simulink subsystem "SMC_mathmatical"  (R2023a)
settings: Solver=VariableStepAuto  StartTime=0.0  StopTime=10.0  RelTol=1e-3
settings Model: Creator=hollis  LastModifiedBy=ethan

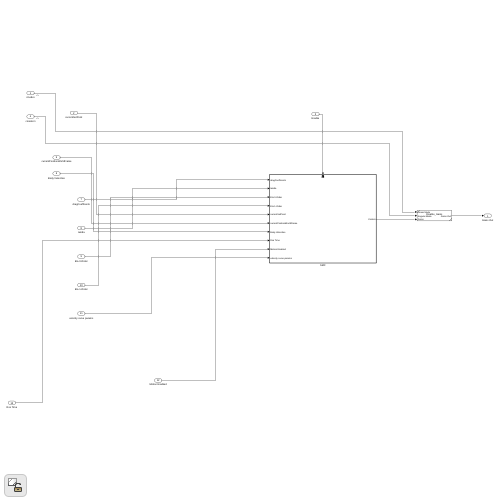
[thumbnail: Simulink's stored preview of the top-level diagram]
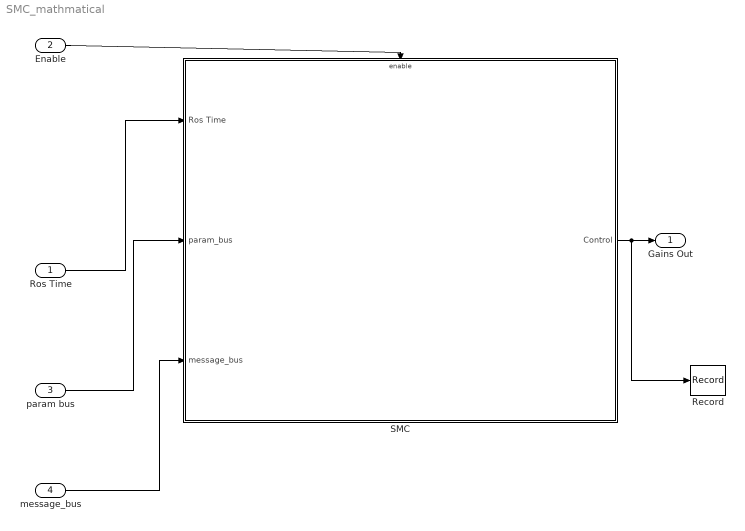
== system SMC_mathmatical ==
  Ros Time : Inport
  Enable : Inport  Port=2
  param bus : Inport  Port=3
  message_bus : Inport  Port=4
  Record : Record  FileSettingsInternal="{\"entries\":[{\"content\":{\"excelSettings\":{\"content\":{},\"type\":\"Streamout.ExcelSettings\"}},\"type\":\"Streamout.FileSettingStorage\",\"uuid\":\"\"}],\"packageUris\":[\"http:\\/\\/schema.mathworks.com\\/mf0\\/streamout_blocks\\/R2020a\"],\"version\":\"1.0\"}"  Layout=[1 1]  SignalsInternal="{\"entries\":[{\"content\":{\"signals\":[{\"content\":{\"blockPath\":[],\"dimensions\":[6],\"domain\":\"\",\"hasChildren\":true,\"lineColor\":\"#22b573\",\"port\":1,\"signalID\":34895,\"signalName\":\"SMC\"},\"type\":\"RecordBlkView.Signal\",\"uuid\":\"\"},{\"content\":{\"blockPath\":[],\"channel\":[1],\"dimensions\":[6],\"domain\":\"\",\"lineColor\":\"#0072bd\",\"parentID\":34895,\"plots\":[1],\"port\":1,\"signalID\":34896,\"signalName\":\"SMC\"},\"type\":\"RecordBlkView.Signal\",\"uuid\":\"\"},{\"content\":{\"blockPath\":[],\"channel\":[2],\"dimensions\":[6],\"domain\":\"\",\"lineColor\":\"#a2142f\",\"parentID\":34895,\"plots\":[1],\"port\":1,\"signalID\":34897,\"signalName\":\"SMC\"},\"type\":\"RecordBlkView.Signal\",\"uuid\":\"\"},{\"content\":{\"blockPath\":[],\"channel\":[3],\"dimensions\":[6],\"domain\":\"\",\"lineColor\":\"#139fff\",\"parentID\":34895,\"plots\":[1],\"port\":1,\"signalID\":34898,\"signalName\":\"SMC\"},\"type\":\"RecordBlkView.Signal\",\"uuid\":\"\"},{\"content\":{\"blockPath\":[],\"channel\":[4],\"dimensions\":[6],\"domain\":\"\",\"lineColor\":\"#ff6929\",\"parentID\":34895,\"plots\":[1],\"port\":1,\"signalID\":34899,\"signalName\":\"SMC\"},\"type\":\"RecordBlkView.Signal\",\"uuid\":\"\"},{\"content\":{\"blockPath\":[],\"channel\":[5],\"dimensions\":[6],\"domain\":\"\",\"lineColor\":\"#b746ff\",\"parentID\":34895,\"plots\":[1],\"port\":1,\"signalID\":34900,\"signalName\":\"SMC\"},\"type\":\"RecordBlkView.Signal\",\"uuid\":\"\"},{\"content\":{\"blockPath\":[],\"channel\":[6],\"dimensions\":[6],\"domain\":\"\",\"lineColor\":\"#64d413\",\"parentID\":34895,\"plots\":[1],\"port\":1,\"signalID\":34901,\"signalName\":\"SMC\"},\"type\":\"RecordBlkView.Signal\",\"uuid\":\"\"}]},\"type\":\"RecordBlkView.InputSignals\",\"uuid\":\"\"}],\"packageUris\":[\"http:\\/\\/schema.mathworks.com\\/mf0\\/streamout_blocks\\/R2020a\"],\"version\":\"1.0\"}"  VisualizationBindings="{\"sparklinesplugin\":{\"info\":[{\"bindingParametersList\":[],\"subplotID\":1}]}}"
  SMC : Subsystem
  Gains Out : Outport
  wires:
  SMC/1(Control) -> Gains Out/1, Record/1
  param bus/1 -> SMC/2(param_bus)
  Ros Time/1 -> SMC/1(Ros Time)
  Enable/1 -> SMC/Enable
  message_bus/1 -> SMC/3(message_bus)

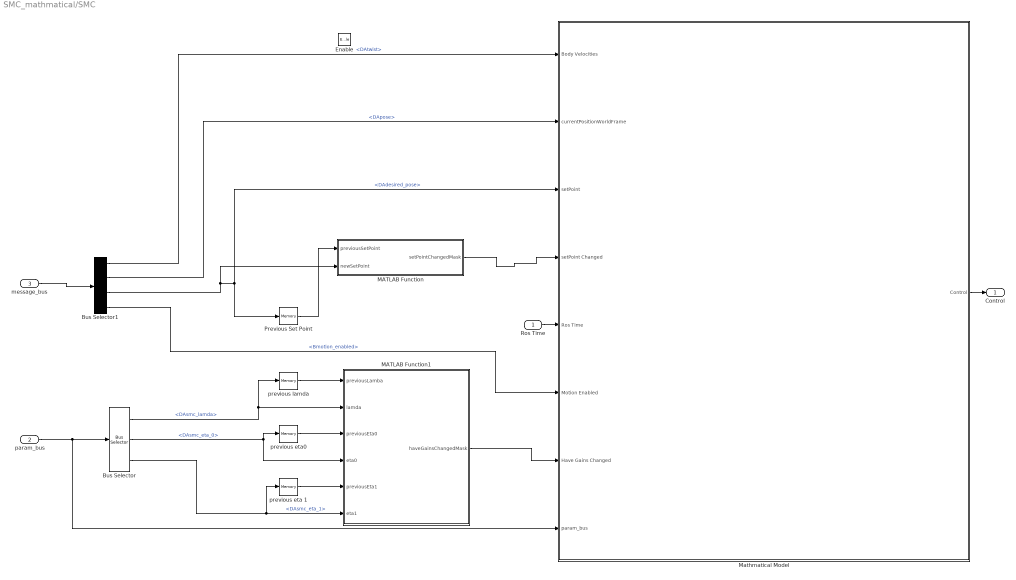
== system SMC_mathmatical/SMC ==
  Ros Time : Inport
  param_bus : Inport  Port=2
  message_bus : Inport  Port=3
  Enable : EnablePort
  Bus Selector : BusSelector  OutputSignals=DAsmc_lamda,DAsmc_eta_0,DAsmc_eta_1
  Bus Selector1 : BusSelector  OutputSignals=current_state.DAtwist,current_state.DApose,desired_pose.DAdesired_pose,Bmotion_enabled
  MATLAB Function : MATLAB Function  TreatAsAtomicUnit=on
  MATLAB Function1 : MATLAB Function  TreatAsAtomicUnit=on
  Mathmatical Model : Subsystem
  Previous Set Point : Memory  InitialCondition=[0,0,0,0,0,0,0]  InheritSampleTime=on
  previous eta 1 : Memory  InheritSampleTime=on
  previous eta0 : Memory  InheritSampleTime=on
  previous lamda : Memory  InheritSampleTime=on
  Control : Outport
  wires:
  Bus Selector1/1 -> Mathmatical Model/1(Body Velocities)  "<DAtwist>"
  Bus Selector1/2 -> Mathmatical Model/2(currentPositionWorldFrame)  "<DApose>"
  message_bus/1 -> Bus Selector1/1
  Bus Selector/3 -> MATLAB Function1/6(eta1), previous eta 1/1  "<DAsmc_eta_1>"
  Bus Selector/2 -> MATLAB Function1/4(eta0), previous eta0/1  "<DAsmc_eta_0>"
  Bus Selector/1 -> MATLAB Function1/2(lamda), previous lamda/1  "<DAsmc_lamda>"
  param_bus/1 -> Mathmatical Model/8(param_bus), Bus Selector/1
  MATLAB Function1/1(haveGainsChangedMask) -> Mathmatical Model/7(Have Gains Changed)
  previous eta 1/1 -> MATLAB Function1/5(previousEta1)
  previous eta0/1 -> MATLAB Function1/3(previousEta0)
  previous lamda/1 -> MATLAB Function1/1(previousLamba)
  Bus Selector1/4 -> Mathmatical Model/6(Motion Enabled)  "<Bmotion_enabled>"
  Ros Time/1 -> Mathmatical Model/5(Ros Time)
  Previous Set Point/1 -> MATLAB Function/1(previousSetPoint)
  MATLAB Function/1(setPointChangedMask) -> Mathmatical Model/4(setPoint Changed)
  Bus Selector1/3 -> Mathmatical Model/3(setPoint), Previous Set Point/1, MATLAB Function/2(newSetPoint)  "<DAdesired_pose>"
  Mathmatical Model/1(Control) -> Control/1

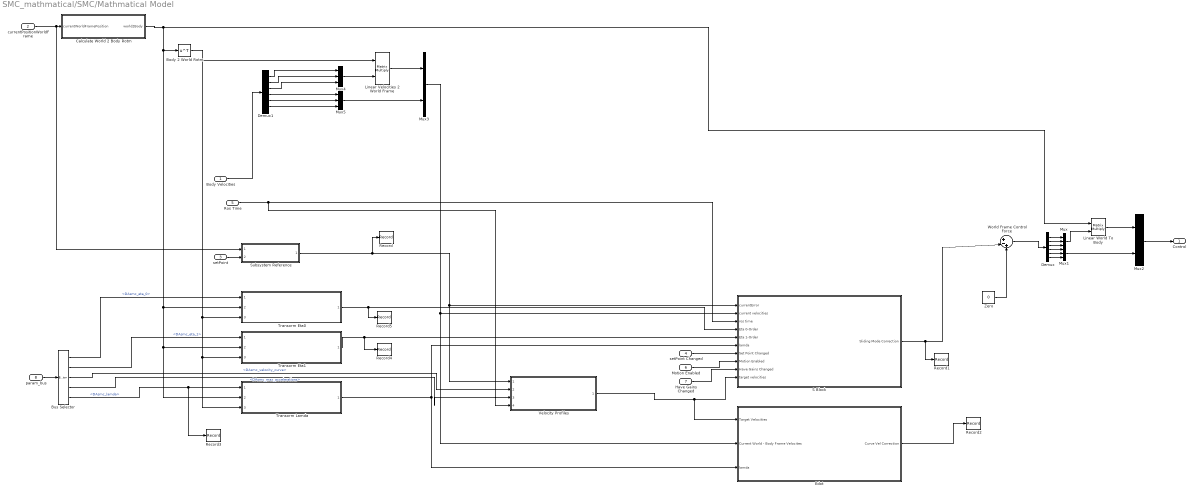
== system SMC_mathmatical/SMC/Mathmatical Model ==
  Body Velocities : Inport
  currentPositionWorldFrame : Inport  Port=2
  setPoint : Inport  Port=3
  setPoint Changed : Inport  Port=4
  Ros Time : Inport  Port=5
  Motion Enabled : Inport  Port=6
  Have Gains Changed : Inport  Port=7
  param_bus : Inport  Port=8
  Body 2 World Rotm : Math  Operator=transpose
  Bus Selector : BusSelector  OutputSignals=DAsmc_eta_0,DAsmc_eta_1,DAsmc_velocity_curve,DAsmc_max_accelerations,DAsmc_lamda
  Calculate World 2 Body Rotm : MATLAB Function  TreatAsAtomicUnit=on
  Demux : Demux  Outputs=6
  Demux1 : Demux  Outputs=6
  Edot : Subsystem
  Linear Velocities 2 World Frame : Product  Multiplication=Matrix(*)
  Linear World To Body : Product  Multiplication=Matrix(*)
  Mux{,1,4..5} (4 alike) : Mux  Inputs=3
  Mux2 : Mux  Inputs=2
  Mux3 : Mux  Inputs=2
  Record : Record  FileSettingsInternal="{\"entries\":[{\"content\":{\"excelSettings\":{\"content\":{},\"type\":\"Streamout.ExcelSettings\"}},\"type\":\"Streamout.FileSettingStorage\",\"uuid\":\"\"}],\"packageUris\":[\"http:\\/\\/schema.mathworks.com\\/mf0\\/streamout_blocks\\/R2020a\"],\"version\":\"1.0\"}"  Layout=[1 1]  SignalsInternal="{\"entries\":[{\"content\":{\"signals\":[{\"content\":{\"blockPath\":[],\"dimensions\":[1,6],\"domain\":\"\",\"hasChildren\":true,\"lineColor\":\"#0072bd\",\"port\":1,\"signalID\":34980,\"signalName\":\"Subsystem Reference\"},\"type\":\"RecordBlkView.Signal\",\"uuid\":\"\"},{\"content\":{\"blockPath\":[],\"channel\":[1,1],\"dimensions\":[1,6],\"domain\":\"\",\"lineColor\":\"#d95319\",\"parentID\":34980,\"plots\":[1],\"port\":1,\"signalID\":34981,\"signalName\":\"Subsystem Reference\"},\"type\":\"RecordBlkView.Signal\",\"uuid\":\"\"},{\"content\":{\"blockPath\":[],\"channel\":[1,2],\"dimensions\":[1,6],\"domain\":\"\",\"lineColor\":\"#b746ff\",\"parentID\":34980,\"plots\":[1],\"port\":1,\"signalID\":34982,\"signalName\":\"Subsystem Reference\"},\"type\":\"RecordBlkView.Signal\",\"uuid\":\"\"},{\"content\":{\"blockPath\":[],\"channel\":[1,3],\"dimensions\":[1,6],\"domain\":\"\",\"lineColor\":\"#64d413\",\"parentID\":34980,\"plots\":[1],\"port\":1,\"signalID\":34983,\"signalName\":\"Subsystem Reference\"},\"type\":\"RecordBlkView.Signal\",\"uuid\":\"\"},{\"content\":{\"blockPath\":[],\"channel\":[1,4],\"dimensions\":[1,6],\"domain\":\"\",\"lineColor\":\"#ff13a6\",\"parentID\":34980,\"plots\":[1],\"port\":1,\"signalID\":34984,\"signalName\":\"Subsystem Reference\"},\"type\":\"RecordBlkView.Signal\",\"uuid\":\"\"},{\"content\":{\"blockPath\":[],\"channel\":[1,5],\"dimensions\":[1,6],\"domain\":\"\",\"lineColor\":\"#fe330a\",\"parentID\":34980,\"plots\":[1],\"port\":1,\"signalID\":34985,\"signalName\":\"Subsystem Reference\"},\"type\":\"RecordBlkView.Signal\",\"uuid\":\"\"},{\"content\":{\"blockPath\":[],\"channel\":[1,6],\"dimensions\":[1,6],\"domain\":\"\",\"lineColor\":\"#22b573\",\"parentID\":34980,\"plots\":[1],\"port\":1,\"signalID\":34986,\"signalName\":\"Subsystem Reference\"},\"type\":\"RecordBlkView.Signal\",\"uuid\":\"\"}]},\"type\":\"RecordBlkView.InputSignals\",\"uuid\":\"\"}],\"packageUris\":[\"http:\\/\\/schema.mathworks.com\\/mf0\\/streamout_blocks\\/R2020a\"],\"version\":\"1.0\"}"  VisualizationBindings="{\"sparklinesplugin\":{\"info\":[{\"bindingParametersList\":[],\"subplotID\":1}]}}"
  Record1 : Record  FileSettingsInternal="{\"entries\":[{\"content\":{\"excelSettings\":{\"content\":{},\"type\":\"Streamout.ExcelSettings\"}},\"type\":\"Streamout.FileSettingStorage\",\"uuid\":\"\"}],\"packageUris\":[\"http:\\/\\/schema.mathworks.com\\/mf0\\/streamout_blocks\\/R2020a\"],\"version\":\"1.0\"}"  Layout=[1 1]  SignalsInternal="{\"entries\":[{\"content\":{\"signals\":[{\"content\":{\"blockPath\":[],\"dimensions\":[6,1],\"domain\":\"\",\"hasChildren\":true,\"lineColor\":\"#22b573\",\"port\":1,\"signalID\":34997,\"signalName\":\"S Block\"},\"type\":\"RecordBlkView.Signal\",\"uuid\":\"\"},{\"content\":{\"blockPath\":[],\"channel\":[1,1],\"dimensions\":[6,1],\"domain\":\"\",\"lineColor\":\"#0072bd\",\"parentID\":34997,\"plots\":[1],\"port\":1,\"signalID\":34998,\"signalName\":\"S Block\"},\"type\":\"RecordBlkView.Signal\",\"uuid\":\"\"},{\"content\":{\"blockPath\":[],\"channel\":[2,1],\"dimensions\":[6,1],\"domain\":\"\",\"lineColor\":\"#4dbeee\",\"parentID\":34997,\"plots\":[1],\"port\":1,\"signalID\":34999,\"signalName\":\"S Block\"},\"type\":\"RecordBlkView.Signal\",\"uuid\":\"\"},{\"content\":{\"blockPath\":[],\"channel\":[3,1],\"dimensions\":[6,1],\"domain\":\"\",\"lineColor\":\"#a2142f\",\"parentID\":34997,\"plots\":[1],\"port\":1,\"signalID\":35000,\"signalName\":\"S Block\"},\"type\":\"RecordBlkView.Signal\",\"uuid\":\"\"},{\"content\":{\"blockPath\":[],\"channel\":[4,1],\"dimensions\":[6,1],\"domain\":\"\",\"lineColor\":\"#139fff\",\"parentID\":34997,\"plots\":[1],\"port\":1,\"signalID\":35001,\"signalName\":\"S Block\"},\"type\":\"RecordBlkView.Signal\",\"uuid\":\"\"},{\"content\":{\"blockPath\":[],\"channel\":[5,1],\"dimensions\":[6,1],\"domain\":\"\",\"lineColor\":\"#ff6929\",\"parentID\":34997,\"plots\":[1],\"port\":1,\"signalID\":35002,\"signalName\":\"S Block\"},\"type\":\"RecordBlkView.Signal\",\"uuid\":\"\"},{\"content\":{\"blockPath\":[],\"channel\":[6,1],\"dimensions\":[6,1],\"domain\":\"\",\"lineColor\":\"#b746ff\",\"parentID\":34997,\"plots\":[1],\"port\":1,\"signalID\":35003,\"signalName\":\"S Block\"},\"type\":\"RecordBlkView.Signal\",\"uuid\":\"\"}]},\"type\":\"RecordBlkView.InputSignals\",\"uuid\":\"\"}],\"packageUris\":[\"http:\\/\\/schema.mathworks.com\\/mf0\\/streamout_blocks\\/R2020a\"],\"version\":\"1.0\"}"  VisualizationBindings="{\"sparklinesplugin\":{\"info\":[{\"bindingParametersList\":[],\"subplotID\":1}]}}"
  Record2 : Record  FileSettingsInternal="{\"entries\":[{\"content\":{\"excelSettings\":{\"content\":{},\"type\":\"Streamout.ExcelSettings\"}},\"type\":\"Streamout.FileSettingStorage\",\"uuid\":\"\"}],\"packageUris\":[\"http:\\/\\/schema.mathworks.com\\/mf0\\/streamout_blocks\\/R2020a\"],\"version\":\"1.0\"}"  Layout=[1 1]  SignalsInternal="{\"entries\":[{\"content\":{\"signals\":[{\"content\":{\"blockPath\":[],\"dimensions\":[6,1],\"domain\":\"\",\"hasChildren\":true,\"lineColor\":\"#d95319\",\"port\":1,\"signalID\":35014,\"signalName\":\"Edot\"},\"type\":\"RecordBlkView.Signal\",\"uuid\":\"\"},{\"content\":{\"blockPath\":[],\"channel\":[1,1],\"dimensions\":[6,1],\"domain\":\"\",\"lineColor\":\"#edb120\",\"parentID\":35014,\"plots\":[1],\"port\":1,\"signalID\":35015,\"signalName\":\"Edot\"},\"type\":\"RecordBlkView.Signal\",\"uuid\":\"\"},{\"content\":{\"blockPath\":[],\"channel\":[2,1],\"dimensions\":[6,1],\"domain\":\"\",\"lineColor\":\"#d95319\",\"parentID\":35014,\"plots\":[1],\"port\":1,\"signalID\":35016,\"signalName\":\"Edot\"},\"type\":\"RecordBlkView.Signal\",\"uuid\":\"\"},{\"content\":{\"blockPath\":[],\"channel\":[3,1],\"dimensions\":[6,1],\"domain\":\"\",\"lineColor\":\"#edb120\",\"parentID\":35014,\"plots\":[1],\"port\":1,\"signalID\":35017,\"signalName\":\"Edot\"},\"type\":\"RecordBlkView.Signal\",\"uuid\":\"\"},{\"content\":{\"blockPath\":[],\"channel\":[4,1],\"dimensions\":[6,1],\"domain\":\"\",\"lineColor\":\"#7e2f8e\",\"parentID\":35014,\"plots\":[1],\"port\":1,\"signalID\":35018,\"signalName\":\"Edot\"},\"type\":\"RecordBlkView.Signal\",\"uuid\":\"\"},{\"content\":{\"blockPath\":[],\"channel\":[5,1],\"dimensions\":[6,1],\"domain\":\"\",\"lineColor\":\"#77ac30\",\"parentID\":35014,\"plots\":[1],\"port\":1,\"signalID\":35019,\"signalName\":\"Edot\"},\"type\":\"RecordBlkView.Signal\",\"uuid\":\"\"},{\"content\":{\"blockPath\":[],\"channel\":[6,1],\"dimensions\":[6,1],\"domain\":\"\",\"lineColor\":\"#4dbeee\",\"parentID\":35014,\"plots\":[1],\"port\":1,\"signalID\":35020,\"signalName\":\"Edot\"},\"type\":\"RecordBlkView.Signal\",\"uuid\":\"\"}]},\"type\":\"RecordBlkView.InputSignals\",\"uuid\":\"\"}],\"packageUris\":[\"http:\\/\\/schema.mathworks.com\\/mf0\\/streamout_blocks\\/R2020a\"],\"version\":\"1.0\"}"  VisualizationBindings="{\"sparklinesplugin\":{\"info\":[{\"bindingParametersList\":[],\"subplotID\":1}]}}"
  Record3 : Record  FileSettingsInternal="{\"entries\":[{\"content\":{\"excelSettings\":{\"content\":{},\"type\":\"Streamout.ExcelSettings\"}},\"type\":\"Streamout.FileSettingStorage\",\"uuid\":\"\"}],\"packageUris\":[\"http:\\/\\/schema.mathworks.com\\/mf0\\/streamout_blocks\\/R2020a\"],\"version\":\"1.0\"}"  Layout=[1 1]  SignalsInternal="{\"entries\":[{\"content\":{\"signals\":[{\"content\":{\"blockPath\":[],\"dimensions\":[1,6],\"domain\":\"\",\"hasChildren\":true,\"lineColor\":\"#b746ff\",\"port\":1,\"signalID\":35031,\"signalName\":\"<DAsmc_lamda>\"},\"type\":\"RecordBlkView.Signal\",\"uuid\":\"\"},{\"content\":{\"blockPath\":[],\"channel\":[1,1],\"dimensions\":[1,6],\"domain\":\"\",\"lineColor\":\"#64d413\",\"parentID\":35031,\"plots\":[1],\"port\":1,\"signalID\":35032,\"signalName\":\"<DAsmc_lamda>\"},\"type\":\"RecordBlkView.Signal\",\"uuid\":\"\"},{\"content\":{\"blockPath\":[],\"channel\":[1,2],\"dimensions\":[1,6],\"domain\":\"\",\"lineColor\":\"#0072bd\",\"parentID\":35031,\"plots\":[1],\"port\":1,\"signalID\":35033,\"signalName\":\"<DAsmc_lamda>\"},\"type\":\"RecordBlkView.Signal\",\"uuid\":\"\"},{\"content\":{\"blockPath\":[],\"channel\":[1,3],\"dimensions\":[1,6],\"domain\":\"\",\"lineColor\":\"#d95319\",\"parentID\":35031,\"plots\":[1],\"port\":1,\"signalID\":35034,\"signalName\":\"<DAsmc_lamda>\"},\"type\":\"RecordBlkView.Signal\",\"uuid\":\"\"},{\"content\":{\"blockPath\":[],\"channel\":[1,4],\"dimensions\":[1,6],\"domain\":\"\",\"lineColor\":\"#edb120\",\"parentID\":35031,\"plots\":[1],\"port\":1,\"signalID\":35035,\"signalName\":\"<DAsmc_lamda>\"},\"type\":\"RecordBlkView.Signal\",\"uuid\":\"\"},{\"content\":{\"blockPath\":[],\"channel\":[1,5],\"dimensions\":[1,6],\"domain\":\"\",\"lineColor\":\"#7e2f8e\",\"parentID\":35031,\"plots\":[1],\"port\":1,\"signalID\":35036,\"signalName\":\"<DAsmc_lamda>\"},\"type\":\"RecordBlkView.Signal\",\"uuid\":\"\"},{\"content\":{\"blockPath\":[],\"channel\":[1,6],\"dimensions\":[1,6],\"domain\":\"\",\"lineColor\":\"#77ac30\",\"parentID\":35031,\"plots\":[1],\"port\":1,\"signalID\":35037,\"signalName\":\"<DAsmc_lamda>\"},\"type\":\"RecordBlkView.Signal\",\"uuid\":\"\"}]},\"type\":\"RecordBlkView.InputSignals\",\"uuid\":\"\"}],\"packageUris\":[\"http:\\/\\/schema.mathworks.com\\/mf0\\/streamout_blocks\\/R2020a\"],\"version\":\"1.0\"}"  VisualizationBindings="{\"sparklinesplugin\":{\"info\":[{\"bindingParametersList\":[],\"subplotID\":1}]}}"
  Record4 : Record  FileSettingsInternal="{\"entries\":[{\"content\":{\"excelSettings\":{\"content\":{},\"type\":\"Streamout.ExcelSettings\"}},\"type\":\"Streamout.FileSettingStorage\",\"uuid\":\"\"}],\"packageUris\":[\"http:\\/\\/schema.mathworks.com\\/mf0\\/streamout_blocks\\/R2020a\"],\"version\":\"1.0\"}"  SignalsInternal="{\"entries\":[{\"content\":{},\"type\":\"RecordBlkView.InputSignals\",\"uuid\":\"\"}],\"packageUris\":[\"http:\\/\\/schema.mathworks.com\\/mf0\\/streamout_blocks\\/R2020a\"],\"version\":\"1.0\"}"  VisualizationBindings="{\"sparklinesplugin\":{\"info\":[{\"bindingParametersList\":[],\"subplotID\":1}]}}"
  Record5 : Record  FileSettingsInternal="{\"entries\":[{\"content\":{\"excelSettings\":{\"content\":{},\"type\":\"Streamout.ExcelSettings\"}},\"type\":\"Streamout.FileSettingStorage\",\"uuid\":\"\"}],\"packageUris\":[\"http:\\/\\/schema.mathworks.com\\/mf0\\/streamout_blocks\\/R2020a\"],\"version\":\"1.0\"}"  SignalsInternal="{\"entries\":[{\"content\":{},\"type\":\"RecordBlkView.InputSignals\",\"uuid\":\"\"}],\"packageUris\":[\"http:\\/\\/schema.mathworks.com\\/mf0\\/streamout_blocks\\/R2020a\"],\"version\":\"1.0\"}"  VisualizationBindings="{\"sparklinesplugin\":{\"info\":[{\"bindingParametersList\":[],\"subplotID\":1}]}}"
  S Block : Subsystem
  Subsystem Reference : Subsystem  ReferencedSubsystem=Normalize_Pose_Error
  Transorm Eta0 : Subsystem  ReferencedSubsystem=Tranfsform_Linear_Gains_To_World
  Transorm Eta1 : Subsystem  ReferencedSubsystem=Tranfsform_Linear_Gains_To_World
  Transorm Lamda : Subsystem  ReferencedSubsystem=Tranfsform_Linear_Gains_To_World
  Velocity Profiles : Subsystem  ReferencedSubsystem=Velocity_Profiles
  World Frame Control Force : Sum  Inputs=|+-+
  Zero : Constant  Value=0  OutDataTypeStr=Inherit: Inherit via back propagation
  Control : Outport
  wires:
  Zero/1 -> World Frame Control Force/3
  Edot/1(Curve Vel Correction) -> Record2/1
  Bus Selector/3 -> Velocity Profiles/2  "<DAsmc_velocity_curve>"
  Bus Selector/4 -> Velocity Profiles/3  "<DAsmc_max_accelerations>"
  Bus Selector/5 -> Transorm Lamda/1, Record3/1  "<DAsmc_lamda>"
  Bus Selector/2 -> Transorm Eta1/1  "<DAsmc_eta_1>"
  Bus Selector/1 -> Transorm Eta0/1  "<DAsmc_eta_0>"
  param_bus/1 -> Bus Selector/1
  Mux3/1 -> Edot/2(Current World - Body Frame Velocites), S Block/2(current velocities)
  Velocity Profiles/1 -> S Block/10(target velocities), Edot/1(Target Velocities)
  Have Gains Changed/1 -> S Block/9(Have Gains Changed)
  Motion Enabled/1 -> S Block/8(Motion Enabled)
  Transorm Eta0/1 -> S Block/4(Eta 0-Order), Record5/1
  Body 2 World Rotm/1 -> Linear Velocities 2 World Frame/1, Transorm Eta0/3, Transorm Eta1/3, Transorm Lamda/3
  setPoint/1 -> Subsystem Reference/2
  Subsystem Reference/1 -> S Block/1(currentError), Velocity Profiles/1, Record/1
  Ros Time/1 -> S Block/3(ros time), Velocity Profiles/4
  setPoint Changed/1 -> S Block/7(Set Point Changed)
  Transorm Eta1/1 -> S Block/5(Eta 1-Order), Record4/1
  Transorm Lamda/1 -> S Block/6(lamda), Edot/3(lamda)
  Mux5/1 -> Mux3/2
  Demux1/6 -> Mux5/3
  Demux1/4 -> Mux5/1
  Demux1/5 -> Mux5/2
  Demux1/3 -> Mux4/3
  Demux1/1 -> Mux4/1
  Demux1/2 -> Mux4/2
  Mux4/1 -> Linear Velocities 2 World Frame/2
  Linear Velocities 2 World Frame/1 -> Mux3/1
  Calculate World 2 Body Rotm/1(world2Body) -> Linear World To Body/1, Transorm Eta0/2, Transorm Eta1/2, Transorm Lamda/2, Body 2 World Rotm/1
  Mux2/1 -> Control/1
  Mux1/1 -> Mux2/2
  Linear World To Body/1 -> Mux2/1
  Mux/1 -> Linear World To Body/2
  Demux/4 -> Mux1/1
  Demux/5 -> Mux1/2
  Demux/6 -> Mux1/3
  Demux/3 -> Mux/3
  Demux/2 -> Mux/2
  Demux/1 -> Mux/1
  World Frame Control Force/1 -> Demux/1
  S Block/1("Sliding Mode Correction ") -> World Frame Control Force/2, Record1/1
  currentPositionWorldFrame/1 -> Calculate World 2 Body Rotm/1(currentWorldFramePosition), Subsystem Reference/1
  Body Velocities/1 -> Demux1/1

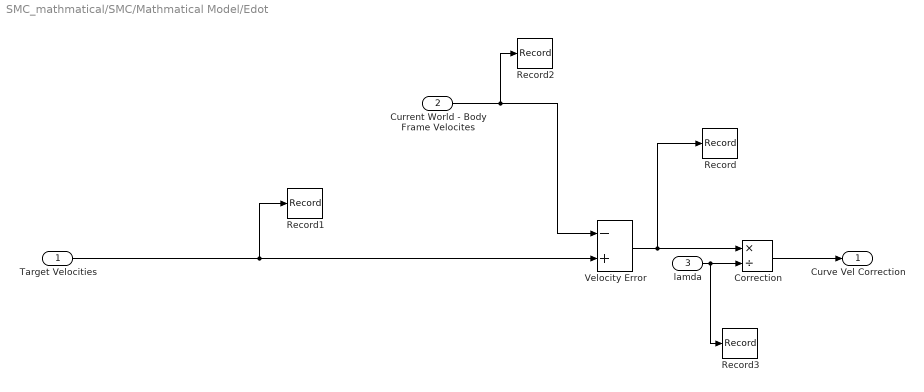
== system SMC_mathmatical/SMC/Mathmatical Model/Edot ==
  Target Velocities : Inport
  Current World - Body Frame Velocites : Inport  Port=2
  lamda : Inport  Port=3
  Correction : Product  Inputs=*/
  Record : Record  FileSettingsInternal="{\"entries\":[{\"content\":{\"excelSettings\":{\"content\":{},\"type\":\"Streamout.ExcelSettings\"}},\"type\":\"Streamout.FileSettingStorage\",\"uuid\":\"\"}],\"packageUris\":[\"http:\\/\\/schema.mathworks.com\\/mf0\\/streamout_blocks\\/R2020a\"],\"version\":\"1.0\"}"  Layout=[1 1]  SignalsInternal="{\"entries\":[{\"content\":{\"signals\":[{\"content\":{\"blockPath\":[],\"dimensions\":[6,1],\"domain\":\"\",\"hasChildren\":true,\"lineColor\":\"#fe330a\",\"port\":1,\"signalID\":34912,\"signalName\":\"Velocity Error\"},\"type\":\"RecordBlkView.Signal\",\"uuid\":\"\"},{\"content\":{\"blockPath\":[],\"channel\":[1,1],\"dimensions\":[6,1],\"domain\":\"\",\"lineColor\":\"#22b573\",\"parentID\":34912,\"plots\":[1],\"port\":1,\"signalID\":34913,\"signalName\":\"Velocity Error\"},\"type\":\"RecordBlkView.Signal\",\"uuid\":\"\"},{\"content\":{\"blockPath\":[],\"channel\":[2,1],\"dimensions\":[6,1],\"domain\":\"\",\"lineColor\":\"#139fff\",\"parentID\":34912,\"plots\":[1],\"port\":1,\"signalID\":34914,\"signalName\":\"Velocity Error\"},\"type\":\"RecordBlkView.Signal\",\"uuid\":\"\"},{\"content\":{\"blockPath\":[],\"channel\":[3,1],\"dimensions\":[6,1],\"domain\":\"\",\"lineColor\":\"#ff6929\",\"parentID\":34912,\"plots\":[1],\"port\":1,\"signalID\":34915,\"signalName\":\"Velocity Error\"},\"type\":\"RecordBlkView.Signal\",\"uuid\":\"\"},{\"content\":{\"blockPath\":[],\"channel\":[4,1],\"dimensions\":[6,1],\"domain\":\"\",\"lineColor\":\"#b746ff\",\"parentID\":34912,\"plots\":[1],\"port\":1,\"signalID\":34916,\"signalName\":\"Velocity Error\"},\"type\":\"RecordBlkView.Signal\",\"uuid\":\"\"},{\"content\":{\"blockPath\":[],\"channel\":[5,1],\"dimensions\":[6,1],\"domain\":\"\",\"lineColor\":\"#64d413\",\"parentID\":34912,\"plots\":[1],\"port\":1,\"signalID\":34917,\"signalName\":\"Velocity Error\"},\"type\":\"RecordBlkView.Signal\",\"uuid\":\"\"},{\"content\":{\"blockPath\":[],\"channel\":[6,1],\"dimensions\":[6,1],\"domain\":\"\",\"lineColor\":\"#ff13a6\",\"parentID\":34912,\"plots\":[1],\"port\":1,\"signalID\":34918,\"signalName\":\"Velocity Error\"},\"type\":\"RecordBlkView.Signal\",\"uuid\":\"\"}]},\"type\":\"RecordBlkView.InputSignals\",\"uuid\":\"\"}],\"packageUris\":[\"http:\\/\\/schema.mathworks.com\\/mf0\\/streamout_blocks\\/R2020a\"],\"version\":\"1.0\"}"  VisualizationBindings="{\"sparklinesplugin\":{\"info\":[{\"bindingParametersList\":[],\"subplotID\":1}]}}"
  Record1 : Record  FileSettingsInternal="{\"entries\":[{\"content\":{\"excelSettings\":{\"content\":{},\"type\":\"Streamout.ExcelSettings\"}},\"type\":\"Streamout.FileSettingStorage\",\"uuid\":\"\"}],\"packageUris\":[\"http:\\/\\/schema.mathworks.com\\/mf0\\/streamout_blocks\\/R2020a\"],\"version\":\"1.0\"}"  Layout=[1 1]  SignalsInternal="{\"entries\":[{\"content\":{\"signals\":[{\"content\":{\"blockPath\":[],\"dimensions\":[6,1],\"domain\":\"\",\"hasChildren\":true,\"lineColor\":\"#0072bd\",\"port\":1,\"signalID\":34929,\"signalName\":\"Target Velocities\"},\"type\":\"RecordBlkView.Signal\",\"uuid\":\"\"},{\"content\":{\"blockPath\":[],\"channel\":[1,1],\"dimensions\":[6,1],\"domain\":\"\",\"lineColor\":\"#d95319\",\"parentID\":34929,\"plots\":[1],\"port\":1,\"signalID\":34930,\"signalName\":\"Target Velocities\"},\"type\":\"RecordBlkView.Signal\",\"uuid\":\"\"},{\"content\":{\"blockPath\":[],\"channel\":[2,1],\"dimensions\":[6,1],\"domain\":\"\",\"lineColor\":\"#7e2f8e\",\"parentID\":34929,\"plots\":[1],\"port\":1,\"signalID\":34931,\"signalName\":\"Target Velocities\"},\"type\":\"RecordBlkView.Signal\",\"uuid\":\"\"},{\"content\":{\"blockPath\":[],\"channel\":[3,1],\"dimensions\":[6,1],\"domain\":\"\",\"lineColor\":\"#77ac30\",\"parentID\":34929,\"plots\":[1],\"port\":1,\"signalID\":34932,\"signalName\":\"Target Velocities\"},\"type\":\"RecordBlkView.Signal\",\"uuid\":\"\"},{\"content\":{\"blockPath\":[],\"channel\":[4,1],\"dimensions\":[6,1],\"domain\":\"\",\"lineColor\":\"#4dbeee\",\"parentID\":34929,\"plots\":[1],\"port\":1,\"signalID\":34933,\"signalName\":\"Target Velocities\"},\"type\":\"RecordBlkView.Signal\",\"uuid\":\"\"},{\"content\":{\"blockPath\":[],\"channel\":[5,1],\"dimensions\":[6,1],\"domain\":\"\",\"lineColor\":\"#a2142f\",\"parentID\":34929,\"plots\":[1],\"port\":1,\"signalID\":34934,\"signalName\":\"Target Velocities\"},\"type\":\"RecordBlkView.Signal\",\"uuid\":\"\"},{\"content\":{\"blockPath\":[],\"channel\":[6,1],\"dimensions\":[6,1],\"domain\":\"\",\"lineColor\":\"#139fff\",\"parentID\":34929,\"plots\":[1],\"port\":1,\"signalID\":34935,\"signalName\":\"Target Velocities\"},\"type\":\"RecordBlkView.Signal\",\"uuid\":\"\"}]},\"type\":\"RecordBlkView.InputSignals\",\"uuid\":\"\"}],\"packageUris\":[\"http:\\/\\/schema.mathworks.com\\/mf0\\/streamout_blocks\\/R2020a\"],\"version\":\"1.0\"}"  VisualizationBindings="{\"sparklinesplugin\":{\"info\":[{\"bindingParametersList\":[],\"subplotID\":1}]}}"
  Record2 : Record  FileSettingsInternal="{\"entries\":[{\"content\":{\"excelSettings\":{\"content\":{},\"type\":\"Streamout.ExcelSettings\"}},\"type\":\"Streamout.FileSettingStorage\",\"uuid\":\"\"}],\"packageUris\":[\"http:\\/\\/schema.mathworks.com\\/mf0\\/streamout_blocks\\/R2020a\"],\"version\":\"1.0\"}"  Layout=[1 1]  SignalsInternal="{\"entries\":[{\"content\":{\"signals\":[{\"content\":{\"blockPath\":[],\"dimensions\":[6],\"domain\":\"\",\"hasChildren\":true,\"lineColor\":\"#edb120\",\"port\":1,\"signalID\":34946,\"signalName\":\"Current World - Body Frame Velocites\"},\"type\":\"RecordBlkView.Signal\",\"uuid\":\"\"},{\"content\":{\"blockPath\":[],\"channel\":[1],\"dimensions\":[6],\"domain\":\"\",\"lineColor\":\"#7e2f8e\",\"parentID\":34946,\"plots\":[1],\"port\":1,\"signalID\":34947,\"signalName\":\"Current World - Body Frame Velocites\"},\"type\":\"RecordBlkView.Signal\",\"uuid\":\"\"},{\"content\":{\"blockPath\":[],\"channel\":[2],\"dimensions\":[6],\"domain\":\"\",\"lineColor\":\"#fe330a\",\"parentID\":34946,\"plots\":[1],\"port\":1,\"signalID\":34948,\"signalName\":\"Current World - Body Frame Velocites\"},\"type\":\"RecordBlkView.Signal\",\"uuid\":\"\"},{\"content\":{\"blockPath\":[],\"channel\":[3],\"dimensions\":[6],\"domain\":\"\",\"lineColor\":\"#22b573\",\"parentID\":34946,\"plots\":[1],\"port\":1,\"signalID\":34949,\"signalName\":\"Current World - Body Frame Velocites\"},\"type\":\"RecordBlkView.Signal\",\"uuid\":\"\"},{\"content\":{\"blockPath\":[],\"channel\":[4],\"dimensions\":[6],\"domain\":\"\",\"lineColor\":\"#0072bd\",\"parentID\":34946,\"plots\":[1],\"port\":1,\"signalID\":34950,\"signalName\":\"Current World - Body Frame Velocites\"},\"type\":\"RecordBlkView.Signal\",\"uuid\":\"\"},{\"content\":{\"blockPath\":[],\"channel\":[5],\"dimensions\":[6],\"domain\":\"\",\"lineColor\":\"#d95319\",\"parentID\":34946,\"plots\":[1],\"port\":1,\"signalID\":34951,\"signalName\":\"Current World - Body Frame Velocites\"},\"type\":\"RecordBlkView.Signal\",\"uuid\":\"\"},{\"content\":{\"blockPath\":[],\"channel\":[6],\"dimensions\":[6],\"domain\":\"\",\"lineColor\":\"#edb120\",\"parentID\":34946,\"plots\":[1],\"port\":1,\"signalID\":34952,\"signalName\":\"Current World - Body Frame Velocites\"},\"type\":\"RecordBlkView.Signal\",\"uuid\":\"\"}]},\"type\":\"RecordBlkView.InputSignals\",\"uuid\":\"\"}],\"packageUris\":[\"http:\\/\\/schema.mathworks.com\\/mf0\\/streamout_blocks\\/R2020a\"],\"version\":\"1.0\"}"  VisualizationBindings="{\"sparklinesplugin\":{\"info\":[{\"bindingParametersList\":[],\"subplotID\":1}]}}"
  Record3 : Record  FileSettingsInternal="{\"entries\":[{\"content\":{\"excelSettings\":{\"content\":{},\"type\":\"Streamout.ExcelSettings\"}},\"type\":\"Streamout.FileSettingStorage\",\"uuid\":\"\"}],\"packageUris\":[\"http:\\/\\/schema.mathworks.com\\/mf0\\/streamout_blocks\\/R2020a\"],\"version\":\"1.0\"}"  Layout=[1 1]  SignalsInternal="{\"entries\":[{\"content\":{\"signals\":[{\"content\":{\"blockPath\":[],\"dimensions\":[6],\"domain\":\"\",\"hasChildren\":true,\"lineColor\":\"#a2142f\",\"port\":1,\"signalID\":34963,\"signalName\":\"lamda\"},\"type\":\"RecordBlkView.Signal\",\"uuid\":\"\"},{\"content\":{\"blockPath\":[],\"channel\":[1],\"dimensions\":[6],\"domain\":\"\",\"lineColor\":\"#139fff\",\"parentID\":34963,\"plots\":[1],\"port\":1,\"signalID\":34964,\"signalName\":\"lamda\"},\"type\":\"RecordBlkView.Signal\",\"uuid\":\"\"},{\"content\":{\"blockPath\":[],\"channel\":[2],\"dimensions\":[6],\"domain\":\"\",\"lineColor\":\"#fe330a\",\"parentID\":34963,\"plots\":[1],\"port\":1,\"signalID\":34965,\"signalName\":\"lamda\"},\"type\":\"RecordBlkView.Signal\",\"uuid\":\"\"},{\"content\":{\"blockPath\":[],\"channel\":[3],\"dimensions\":[6],\"domain\":\"\",\"lineColor\":\"#22b573\",\"parentID\":34963,\"plots\":[1],\"port\":1,\"signalID\":34966,\"signalName\":\"lamda\"},\"type\":\"RecordBlkView.Signal\",\"uuid\":\"\"},{\"content\":{\"blockPath\":[],\"channel\":[4],\"dimensions\":[6],\"domain\":\"\",\"lineColor\":\"#0072bd\",\"parentID\":34963,\"plots\":[1],\"port\":1,\"signalID\":34967,\"signalName\":\"lamda\"},\"type\":\"RecordBlkView.Signal\",\"uuid\":\"\"},{\"content\":{\"blockPath\":[],\"channel\":[5],\"dimensions\":[6],\"domain\":\"\",\"lineColor\":\"#d95319\",\"parentID\":34963,\"plots\":[1],\"port\":1,\"signalID\":34968,\"signalName\":\"lamda\"},\"type\":\"RecordBlkView.Signal\",\"uuid\":\"\"},{\"content\":{\"blockPath\":[],\"channel\":[6],\"dimensions\":[6],\"domain\":\"\",\"lineColor\":\"#edb120\",\"parentID\":34963,\"plots\":[1],\"port\":1,\"signalID\":34969,\"signalName\":\"lamda\"},\"type\":\"RecordBlkView.Signal\",\"uuid\":\"\"}]},\"type\":\"RecordBlkView.InputSignals\",\"uuid\":\"\"}],\"packageUris\":[\"http:\\/\\/schema.mathworks.com\\/mf0\\/streamout_blocks\\/R2020a\"],\"version\":\"1.0\"}"  VisualizationBindings="{\"sparklinesplugin\":{\"info\":[{\"bindingParametersList\":[],\"subplotID\":1}]}}"
  Velocity Error : Sum  Inputs=-+
  Curve Vel Correction : Outport
  wires:
  Target Velocities/1 -> Velocity Error/2, Record1/1
  Velocity Error/1 -> Correction/1, Record/1
  Current World - Body Frame Velocites/1 -> Velocity Error/1, Record2/1
  lamda/1 -> Correction/2, Record3/1
  Correction/1 -> Curve Vel Correction/1

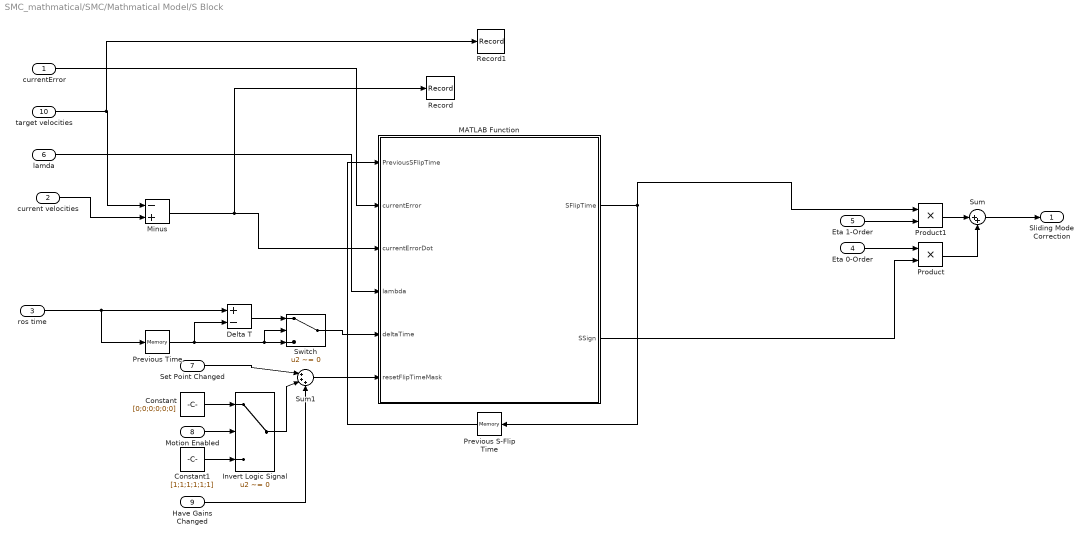
== system SMC_mathmatical/SMC/Mathmatical Model/S Block ==
  currentError : Inport
  current velocities : Inport  Port=2
  ros time : Inport  Port=3
  Eta 0-Order : Inport  Port=4
  Eta 1-Order : Inport  Port=5
  lamda : Inport  Port=6
  Set Point Changed : Inport  Port=7
  Motion Enabled : Inport  Port=8
  Have Gains Changed : Inport  Port=9
  target velocities : Inport  Port=10
  Constant : Constant  Value=[0;0;0;0;0;0]
  Constant1 : Constant  Value=[1;1;1;1;1;1]
  Delta T : Sum  Inputs=+-
  Invert Logic Signal : Switch  Criteria=u2 ~= 0  SaturateOnIntegerOverflow=off  InputSameDT=off
  MATLAB Function : MATLAB Function  TreatAsAtomicUnit=on
  Minus : Sum  Inputs=-+
  Previous S-Flip Time : Memory  InitialCondition=[0;0;0;0;0;0]  InheritSampleTime=on
  Previous Time : Memory  InheritSampleTime=on
  Product : Product
  Product1 : Product
  Record : Record  FileSettingsInternal="{\"entries\":[{\"content\":{\"excelSettings\":{\"content\":{},\"type\":\"Streamout.ExcelSettings\"}},\"type\":\"Streamout.FileSettingStorage\",\"uuid\":\"\"}],\"packageUris\":[\"http:\\/\\/schema.mathworks.com\\/mf0\\/streamout_blocks\\/R2020a\"],\"version\":\"1.0\"}"  Layout=[1 1]  SignalsInternal="{\"entries\":[{\"content\":{\"signals\":[{\"content\":{\"blockPath\":[],\"dimensions\":[6,1],\"domain\":\"\",\"hasChildren\":true,\"lineColor\":\"#b746ff\",\"port\":1,\"signalID\":35048,\"signalName\":\"Minus\"},\"type\":\"RecordBlkView.Signal\",\"uuid\":\"\"},{\"content\":{\"blockPath\":[],\"channel\":[1,1],\"dimensions\":[6,1],\"domain\":\"\",\"lineColor\":\"#64d413\",\"parentID\":35048,\"plots\":[1],\"port\":1,\"signalID\":35049,\"signalName\":\"Minus\"},\"type\":\"RecordBlkView.Signal\",\"uuid\":\"\"},{\"content\":{\"blockPath\":[],\"channel\":[2,1],\"dimensions\":[6,1],\"domain\":\"\",\"lineColor\":\"#ff6929\",\"parentID\":35048,\"plots\":[1],\"port\":1,\"signalID\":35050,\"signalName\":\"Minus\"},\"type\":\"RecordBlkView.Signal\",\"uuid\":\"\"},{\"content\":{\"blockPath\":[],\"channel\":[3,1],\"dimensions\":[6,1],\"domain\":\"\",\"lineColor\":\"#b746ff\",\"parentID\":35048,\"plots\":[1],\"port\":1,\"signalID\":35051,\"signalName\":\"Minus\"},\"type\":\"RecordBlkView.Signal\",\"uuid\":\"\"},{\"content\":{\"blockPath\":[],\"channel\":[4,1],\"dimensions\":[6,1],\"domain\":\"\",\"lineColor\":\"#64d413\",\"parentID\":35048,\"port\":1,\"signalID\":35052,\"signalName\":\"Minus\"},\"type\":\"RecordBlkView.Signal\",\"uuid\":\"\"},{\"content\":{\"blockPath\":[],\"channel\":[5,1],\"dimensions\":[6,1],\"domain\":\"\",\"lineColor\":\"#ff13a6\",\"parentID\":35048,\"port\":1,\"signalID\":35053,\"signalName\":\"Minus\"},\"type\":\"RecordBlkView.Signal\",\"uuid\":\"\"},{\"content\":{\"blockPath\":[],\"channel\":[6,1],\"dimensions\":[6,1],\"domain\":\"\",\"lineColor\":\"#fe330a\",\"parentID\":35048,\"port\":1,\"signalID\":35054,\"signalName\":\"Minus\"},\"type\":\"RecordBlkView.Signal\",\"uuid\":\"\"}]},\"type\":\"RecordBlkView.InputSignals\",\"uuid\":\"\"}],\"packageUris\":[\"http:\\/\\/schema.mathworks.com\\/mf0\\/streamout_blocks\\/R2020a\"],\"version\":\"1.0\"}"  VisualizationBindings="{\"sparklinesplugin\":{\"info\":[{\"bindingParametersList\":[],\"subplotID\":1}]}}"
  Record1 : Record  FileSettingsInternal="{\"entries\":[{\"content\":{\"excelSettings\":{\"content\":{},\"type\":\"Streamout.ExcelSettings\"}},\"type\":\"Streamout.FileSettingStorage\",\"uuid\":\"\"}],\"packageUris\":[\"http:\\/\\/schema.mathworks.com\\/mf0\\/streamout_blocks\\/R2020a\"],\"version\":\"1.0\"}"  Layout=[1 1]  SignalsInternal="{\"entries\":[{\"content\":{\"signals\":[{\"content\":{\"blockPath\":[],\"dimensions\":[6,1],\"domain\":\"\",\"hasChildren\":true,\"lineColor\":\"#d95319\",\"port\":1,\"signalID\":35065,\"signalName\":\"target velocities\"},\"type\":\"RecordBlkView.Signal\",\"uuid\":\"\"},{\"content\":{\"blockPath\":[],\"channel\":[1,1],\"dimensions\":[6,1],\"domain\":\"\",\"lineColor\":\"#edb120\",\"parentID\":35065,\"plots\":[1],\"port\":1,\"signalID\":35066,\"signalName\":\"target velocities\"},\"type\":\"RecordBlkView.Signal\",\"uuid\":\"\"},{\"content\":{\"blockPath\":[],\"channel\":[2,1],\"dimensions\":[6,1],\"domain\":\"\",\"lineColor\":\"#4dbeee\",\"parentID\":35065,\"port\":1,\"signalID\":35067,\"signalName\":\"target velocities\"},\"type\":\"RecordBlkView.Signal\",\"uuid\":\"\"},{\"content\":{\"blockPath\":[],\"channel\":[3,1],\"dimensions\":[6,1],\"domain\":\"\",\"lineColor\":\"#a2142f\",\"parentID\":35065,\"port\":1,\"signalID\":35068,\"signalName\":\"target velocities\"},\"type\":\"RecordBlkView.Signal\",\"uuid\":\"\"},{\"content\":{\"blockPath\":[],\"channel\":[4,1],\"dimensions\":[6,1],\"domain\":\"\",\"lineColor\":\"#139fff\",\"parentID\":35065,\"port\":1,\"signalID\":35069,\"signalName\":\"target velocities\"},\"type\":\"RecordBlkView.Signal\",\"uuid\":\"\"},{\"content\":{\"blockPath\":[],\"channel\":[5,1],\"dimensions\":[6,1],\"domain\":\"\",\"lineColor\":\"#ff6929\",\"parentID\":35065,\"port\":1,\"signalID\":35070,\"signalName\":\"target velocities\"},\"type\":\"RecordBlkView.Signal\",\"uuid\":\"\"},{\"content\":{\"blockPath\":[],\"channel\":[6,1],\"dimensions\":[6,1],\"domain\":\"\",\"lineColor\":\"#b746ff\",\"parentID\":35065,\"port\":1,\"signalID\":35071,\"signalName\":\"target velocities\"},\"type\":\"RecordBlkView.Signal\",\"uuid\":\"\"}]},\"type\":\"RecordBlkView.InputSignals\",\"uuid\":\"\"}],\"packageUris\":[\"http:\\/\\/schema.mathworks.com\\/mf0\\/streamout_blocks\\/R2020a\"],\"version\":\"1.0\"}"  VisualizationBindings="{\"sparklinesplugin\":{\"info\":[{\"bindingParametersList\":[],\"subplotID\":1}]}}"
  Sum : Sum  Inputs=|++
  Sum1 : Sum  Inputs=|+++
  Switch : Switch  Criteria=u2 ~= 0  SaturateOnIntegerOverflow=off  InputSameDT=off
  "Sliding Mode Correction " : Outport
  wires:
  Minus/1 -> MATLAB Function/3(currentErrorDot), Record/1
  current velocities/1 -> Minus/2
  target velocities/1 -> Minus/1, Record1/1
  Invert Logic Signal/1 -> Sum1/2
  Have Gains Changed/1 -> Sum1/3
  Delta T/1 -> Switch/1
  Switch/1 -> MATLAB Function/5(deltaTime)
  ros time/1 -> Delta T/1, Previous Time/1
  Previous Time/1 -> Delta T/2, Switch/3, Switch/2
  Constant1/1 -> Invert Logic Signal/3
  Constant/1 -> Invert Logic Signal/1
  Motion Enabled/1 -> Invert Logic Signal/2
  Set Point Changed/1 -> Sum1/1
  Sum1/1 -> MATLAB Function/6(resetFlipTimeMask)
  lamda/1 -> MATLAB Function/4(lambda)
  Eta 1-Order/1 -> Product1/2
  Eta 0-Order/1 -> Product/1
  Previous S-Flip Time/1 -> MATLAB Function/1(PreviousSFlipTime)
  Sum/1 -> "Sliding Mode Correction "/1
  MATLAB Function/1(SFlipTime) -> Previous S-Flip Time/1, Product1/1
  Product1/1 -> Sum/1
  Product/1 -> Sum/2
  currentError/1 -> MATLAB Function/2(currentError)
  MATLAB Function/2(SSign) -> Product/2

== matlab function SMC_mathmatical/SMC/MATLAB Function ==
  data: previousSetPoint input; setPointChangedMask output; newSetPoint input
function setPointChangedMask = fcn(previousSetPoint, newSetPoint)

setPointChangedMask = zeros(1,6);

%determine wether or not the set point has chnaged - element wise

previousEulerSetPoint = [previousSetPoint(1), previousSetPoint(2), previousSetPoint(3), quat2eul([previousSetPoint(7), previousSetPoint(4), previousSetPoint(5), previousSetPoint(6)])];
newEulerSetPoint = [newSetPoint(1), newSetPoint(2), newSetPoint(3), quat2eul([newSetPoint(7), newSetPoint(4), newSetPoint(5), newSetPoint(6)])];

%not changed = 0, true - everything else
setPointChangedMask = abs(previousEulerSetPoint - newEulerSetPoint);

%allow buffer on angular to account for slight shift due to conversion
%error...
for i=4:6
    if(setPointChangedMask(i) < .1)
        setPointChangedMask(i) = 0;
    end

    %catch nans and reset if they occur
    if(isnan(setPointChangedMask(i)))
        setPointChangedMask(i) = 1;
    end
end

== matlab function SMC_mathmatical/SMC/MATLAB Function1 ==
  data: previousLamba input; haveGainsChangedMask output; lamda input; previousEta0 input; eta0 input; previousEta1 input; eta1 input
function haveGainsChangedMask = fcn(previousLamba, lamda, previousEta0, eta0, previousEta1, eta1)

%determine wether or not the set point has chnaged element wise
haveGainsChangedMask = abs(previousLamba - lamda) + abs(previousEta0 - eta0) + abs(previousEta1 - eta1);

== matlab function SMC_mathmatical/SMC/Mathmatical Model/Calculate World 2 Body Rotm ==
  data: currentWorldFramePosition input; world2Body output
function world2Body = fcn(currentWorldFramePosition)

%convert ros2 quat to matlab quat - quat is last 
quat = [currentWorldFramePosition(7), currentWorldFramePosition(4), currentWorldFramePosition(5), currentWorldFramePosition(6)];

%calculate the rotation matrix representing the current orientation
world2Body = quat2rotm(quat);

%matlab issue
world2Body = transpose(world2Body);

== matlab function SMC_mathmatical/SMC/Mathmatical Model/S Block/MATLAB Function ==
  data: PreviousSFlipTime input; SFlipTime output; currentError input; currentErrorDot input; lambda input; deltaTime input; SSign output; resetFlipTimeMask input
function [SFlipTime, SSign] = fcn(PreviousSFlipTime, currentError, currentErrorDot, lambda, deltaTime, resetFlipTimeMask)

%FlipTime, SSign and Previous are 6 by arrays - 1 per dof

SFlipTime = PreviousSFlipTime;
SSign = zeros(6,1);

%calculate S
S = currentError + lambda' .* currentErrorDot';


%just so nothing explodes - ill be impressed if this happens
for i=1:6

    %ensure no S equals zero
    if(S(i) == 0)
        SSign(i) = 0;
    else
        SSign(i) = S(i) / abs(S(i));
    end
end


%see if Sdot has flipped
for i=1:6

    %if the flip time is not to be reset
    if(~resetFlipTimeMask(i))
        if(SFlipTime(i) * SSign(i) > 0)
            SFlipTime(i) = SFlipTime(i) + deltaTime * SSign(i);
        else
            SFlipTime(i) = deltaTime * SSign(i);
        end
    else
       SFlipTime(i) = 0;
    end
end
